simulink model "Python_GPUtesting_noPS"  (R2019a)
settings: Solver=FixedStepAuto  StartTime=0.0  StopTime=inf  FixedStep=1/ModelRate  RelTol=1e-3  EnableMultiTasking=on
undefined symbols (not defined in the file): DataRate, ModelRate, Ratio
libraries: xpcrtudplib x6, slrtlib x6, etargetslib x4
settings Model: SimulationMode=external  Creator=xugx0  LastModifiedBy=SI
settings SolverCC: ConcurrentTasks=on  AutoInsertRateTranBlk=on
settings DataIOCC: SaveFormat=StructureWithTime
settings OptimizationCC: BlockReduction=off  OptimizeBlockIOStorage=off  BufferReuse=off  GlobalBufferReuse=off  ExpressionFolding=off  LocalBlockOutputs=off  OptimizeDataStoreBuffers=off  BusAssignmentInplaceUpdate=off
settings DebuggingCC: ArithmeticOperatorsInVariantConditions=warning
settings HardwareCC: ProdBitPerPointer=32  ProdBitPerSizeT=32  ProdBitPerPtrDiffT=32  ProdLargestAtomicFloat=None  ProdWordSize=32  ProdLongLongMode=on  ProdHWDeviceType=Generic->32-bit x86 compatible
settings RTWCC: SystemTargetFile=slrt.tlc  TemplateMakefile=slrt_default_tmf  Description=Simulink Real-Time  CodeExecutionProfiling=on  RTWCompilerOptimization=on
settings CodeAppCC: StateflowObjectComments=on
settings SimulinkRealTimeCC: SupportVariableSizeSignals=on  PreserveStateflowLocalDataDimensions=off  RL32LogTETModifier=off  xPCConcurrentTasks=on

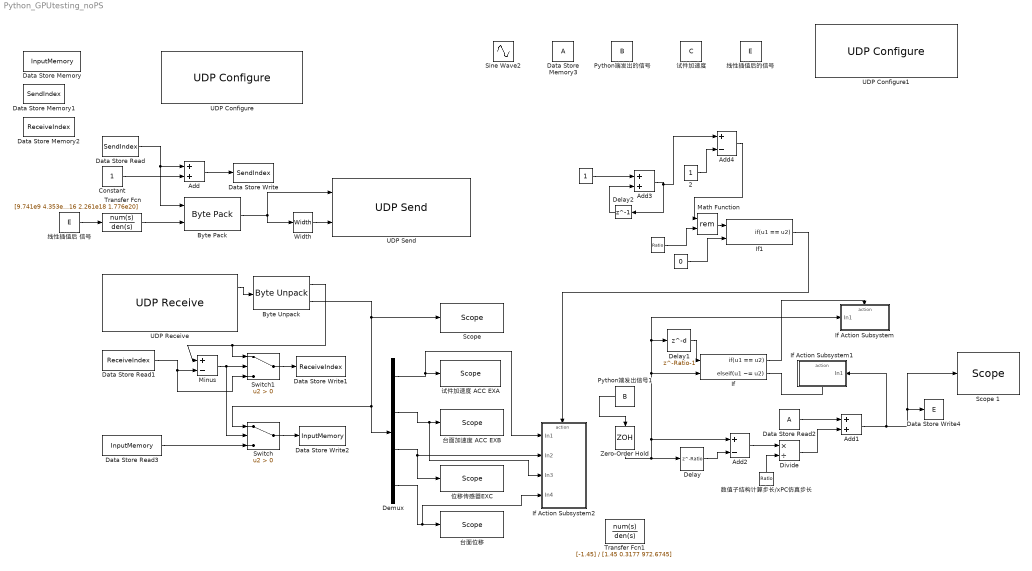
== system Python_GPUtesting_noPS ==
  " " : Constant  Value=Ratio
  " " : Constant  Value=0
  " " : Constant
  " 2" : Constant
  Add : Sum
  Add1 : Sum
  Add2 : Sum  Inputs=+-
  Add3 : Sum
  Add4 : Sum  Inputs=+-
  Byte Pack : etargetslib/Byte Pack  datatypes={'uint32','double'}  byteAlign=1
      settings: SourceProductName=MATLAB Coder
  Byte Unpack : etargetslib/Byte Unpack  dimensions={[1],[NumberOfInputSignals]}  datatypes={'uint32','double'}  byteAlign=1
      settings: SourceProductName=MATLAB Coder
  Constant : Constant  OutDataTypeStr=uint32
  Data Store Memory : DataStoreMemory  DataStoreName=InputMemory  ReadBeforeWriteMsg=warning  WriteAfterWriteMsg=warning  WriteAfterReadMsg=warning  InitialValue=InputMemInitV  ShowAdditionalParam=off
  Data Store Memory1 : DataStoreMemory  DataStoreName=SendIndex  ReadBeforeWriteMsg=warning  WriteAfterWriteMsg=warning  WriteAfterReadMsg=warning  ShowAdditionalParam=off  OutDataTypeStr=uint32
  Data Store Memory2 : DataStoreMemory  DataStoreName=ReceiveIndex  ReadBeforeWriteMsg=warning  WriteAfterWriteMsg=warning  WriteAfterReadMsg=warning  ShowAdditionalParam=off  OutDataTypeStr=uint32
  Data Store Memory3 : DataStoreMemory  ReadBeforeWriteMsg=warning  WriteAfterWriteMsg=warning  WriteAfterReadMsg=warning  ShowAdditionalParam=off
  Data Store Read : DataStoreRead  DataStoreName=SendIndex
  Data Store Read1 : DataStoreRead  DataStoreName=ReceiveIndex
  Data Store Read2 : DataStoreRead
  Data Store Read3 : DataStoreRead  DataStoreName=InputMemory
  Data Store Write : DataStoreWrite  DataStoreName=SendIndex
  Data Store Write1 : DataStoreWrite  DataStoreName=ReceiveIndex
  Data Store Write2 : DataStoreWrite  DataStoreName=InputMemory
  Data Store Write4 : DataStoreWrite  DataStoreName=E
  Delay : Delay  DelayLength=Ratio  InitialCondition=0
  Delay1 : Delay  DelayLength=Ratio-1  InitialCondition=0
  Delay2 : Delay  DelayLength=1  InitialCondition=0
  Demux : Demux
  Divide : Product  Inputs=*/
  If : If  NumInputs=2  IfExpression=u1 == u2  ElseIfExpressions=u1 ~= u2  ShowElse=off
  If Action Subsystem : Subsystem  TreatAsAtomicUnit=on
  If Action Subsystem1 : Subsystem  TreatAsAtomicUnit=on
  If Action Subsystem2 : Subsystem  TreatAsAtomicUnit=on
  If1 : If  NumInputs=2  IfExpression=u1 == u2  ShowElse=off
  Math Function : Math  Operator=rem  SaturateOnIntegerOverflow=on
  Minus : Sum  Inputs=+-
  Python端发出信号1 : DataStoreRead  DataStoreName=B
  Python端发出的信号 : DataStoreMemory  DataStoreName=B  ReadBeforeWriteMsg=warning  WriteAfterWriteMsg=warning  WriteAfterReadMsg=warning  ShowAdditionalParam=off
  "Scope " : slrtlib/Displays and Logging/Scope   scopeno=1  scopetype=Target  autostart=on  viewmode=Graphical sliding  formatstr='%15.6f'  grid=on  ylimits=[0,0]  nosamples=4000  noprepostsamples=0  interleave=1  triggermode=FreeRun  triggersignal=1  trigsignalfromport=off  triggerlevel=0.0  triggerslope=Either  triggerscope=1  triggersample=0  filename=data.dat  mode=Lazy  writesize=512  autorestart=off  dynamicfilemode=off  maxwritefilesize=512*1024^2
  Scope 1 : slrtlib/Displays and Logging/Scope   scopeno=2  scopetype=Target  autostart=on  viewmode=Graphical sliding  formatstr='%15.6f'  grid=on  ylimits=[0,0]  nosamples=4000  noprepostsamples=0  interleave=1  triggermode=FreeRun  triggersignal=1  trigsignalfromport=off  triggerlevel=0.0  triggerslope=Either  triggerscope=1  triggersample=0  filename=data.dat  mode=Lazy  writesize=512  autorestart=off  dynamicfilemode=off  maxwritefilesize=512*1024^2
  Sine Wave2 : Sin  Frequency=10  SampleTime=1/ModelRate
  Switch : Switch  Criteria=u2 > Threshold
  Switch1 : Switch  Criteria=u2 > Threshold
  Transfer Fcn : TransferFcn  Numerator=[9.741e9 4.353e13 1.087e16 2.844e18 1.773e20]  Denominator=[1.823e10 2.291e13 1.08e16 2.261e18 1.776e20]
  Transfer Fcn1 : TransferFcn  Numerator=[-1.45]  Denominator=[1.45 0.3177 972.6745]
  UDP Configure : xpcrtudplib/UDP Configure  Priority=-1  IpAddress=169.254.86.80  SubnetMask=255.255.0.0  Gateway=0.0.0.0  PciBus=5  PciSlot=Slot  PciFunction=0  ID=1  tune=0  disable=off  enableMulticast=off  MulticastIpAddress={}  MulticastMask={}
      settings: SourceProductName=Simulink Real-Time  SourceProductBaseCode=XP
  UDP Configure1 : xpcrtudplib/UDP Configure  Priority=-1  IpAddress=192.168.0.100  SubnetMask=255.255.255.0  Gateway=0.0.0.0  PciBus=4  PciSlot=Slot  PciFunction=0  ID=1  tune=0  disable=off  enableMulticast=off  MulticastIpAddress={}  MulticastMask={}
      settings: SourceProductName=Simulink Real-Time  SourceProductBaseCode=XP
  UDP Receive : xpcrtudplib/UDP Receive  ipAddressVal=169.254.86.80  localPort=LocalPort  rcvWidth=receiveLength  rcvFmAny=off  fmAddress=169.254.86.81  rcvMulticast=off  multicastAddress={}  maxUDPQueue=8  sampleTime=1/DataRate
      settings: SourceProductName=Simulink Real-Time
  UDP Send : xpcrtudplib/UDP Send  ipAddressVal=169.254.86.80  localPort=-1  toAddress=169.254.86.81  toPort=RemotePort  sampleTime=1/DataRate
      settings: SourceProductName=Simulink Real-Time  SourceProductBaseCode=XP
  Width : Width
  Zero-Order Hold : ZeroOrderHold  SampleTime=1/ModelRate
  位移传感器EXC : slrtlib/Displays and Logging/Scope   scopeno=6  scopetype=Target  autostart=on  viewmode=Graphical sliding  formatstr='%15.6f'  grid=on  ylimits=[0,0]  nosamples=4000  noprepostsamples=0  interleave=1  triggermode=FreeRun  triggersignal=1  trigsignalfromport=off  triggerlevel=0.0  triggerslope=Either  triggerscope=1  triggersample=0  filename=data.dat  mode=Lazy  writesize=512  autorestart=off  dynamicfilemode=off  maxwritefilesize=512*1024^2
  台面位移 : slrtlib/Displays and Logging/Scope   scopeno=7  scopetype=Target  autostart=on  viewmode=Graphical sliding  formatstr='%15.6f'  grid=on  ylimits=[0,0]  nosamples=4000  noprepostsamples=0  interleave=1  triggermode=FreeRun  triggersignal=1  trigsignalfromport=off  triggerlevel=0.0  triggerslope=Either  triggerscope=1  triggersample=0  filename=data.dat  mode=Lazy  writesize=512  autorestart=off  dynamicfilemode=off  maxwritefilesize=512*1024^2
  台面加速度 ACC EXB : slrtlib/Displays and Logging/Scope   scopeno=5  scopetype=Target  autostart=on  viewmode=Graphical sliding  formatstr='%15.6f'  grid=on  ylimits=[0,0]  nosamples=4000  noprepostsamples=0  interleave=1  triggermode=FreeRun  triggersignal=1  trigsignalfromport=off  triggerlevel=0.0  triggerslope=Either  triggerscope=1  triggersample=0  filename=data.dat  mode=Lazy  writesize=512  autorestart=off  dynamicfilemode=off  maxwritefilesize=512*1024^2
  数值子结构计算步长/xPC仿真步长 : Constant  Value=Ratio
  线性插值后 信号 : DataStoreRead  DataStoreName=E
  线性插值后的信号 : DataStoreMemory  DataStoreName=E  ReadBeforeWriteMsg=warning  WriteAfterWriteMsg=warning  WriteAfterReadMsg=warning  ShowAdditionalParam=off
  试件加速度 : DataStoreMemory  DataStoreName=C  ReadBeforeWriteMsg=warning  WriteAfterWriteMsg=warning  WriteAfterReadMsg=warning  ShowAdditionalParam=off
  试件加速度 ACC EXA : slrtlib/Displays and Logging/Scope   scopeno=4  scopetype=Target  autostart=on  viewmode=Graphical sliding  formatstr='%15.6f'  grid=on  ylimits=[0,0]  nosamples=4000  noprepostsamples=0  interleave=1  triggermode=FreeRun  triggersignal=1  trigsignalfromport=off  triggerlevel=0.0  triggerslope=Either  triggerscope=1  triggersample=0  filename=data.dat  mode=Lazy  writesize=512  autorestart=off  dynamicfilemode=off  maxwritefilesize=512*1024^2
  wires:
  Byte Pack/1 -> UDP Send/1, Width/1
  Width/1 -> UDP Send/2
  Switch/1 -> Data Store Write2/1
  Add/1 -> Data Store Write/1
  Constant/1 -> Add/2
  Data Store Read/1 -> Add/1, Byte Pack/1
  Minus/1 -> Switch1/2, Switch/2
  Data Store Read3/1 -> Switch/3
  UDP Receive/1 -> Byte Unpack/1
  Byte Unpack/1 -> Minus/1, Switch1/1
  Data Store Read1/1 -> Minus/2, Switch1/3
  Switch1/1 -> Data Store Write1/1
  Byte Unpack/2 -> Switch/1, Demux/1, "Scope "/1
  Add1/1 -> Scope 1/1, Data Store Write4/1, If Action Subsystem1/1(In1)
  Add2/1 -> Divide/1
  数值子结构计算步长/xPC仿真步长/1 -> Divide/2
  Divide/1 -> Add1/2
  Delay/1 -> Add2/2
  If/1 -> If Action Subsystem/Action
  If/2 -> If Action Subsystem1/Action
  Data Store Read2/1 -> Add1/1
  Zero-Order Hold/1 -> Add2/1, If/2, Delay1/1, If Action Subsystem/1(In1), Delay/1
  Delay1/1 -> If/1
  Python端发出信号1/1 -> Zero-Order Hold/1
  " "/1 -> Add3/1
  If1/1 -> If Action Subsystem2/Action
  Math Function/1 -> If1/1
  " "/1 -> Math Function/2
  " "/1 -> If1/2
  Add3/1 -> Add4/1, Delay2/1
  Delay2/1 -> Add3/2
  Demux/1 -> If Action Subsystem2/1(In1), 试件加速度 ACC EXA/1
  " 2"/1 -> Add4/2
  Add4/1 -> Math Function/1
  Demux/2 -> If Action Subsystem2/3(In3), 台面加速度 ACC EXB/1
  Demux/3 -> 位移传感器EXC/1, If Action Subsystem2/2(In2)
  Demux/4 -> If Action Subsystem2/4(In4), 台面位移/1
  Transfer Fcn/1 -> Byte Pack/2
  线性插值后 信号/1 -> Transfer Fcn/1

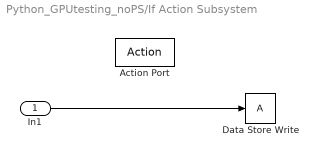
== system Python_GPUtesting_noPS/If Action Subsystem ==
  In1 : Inport
  Action Port : ActionPort  ActionPortLabel=if(u1 == u2)
  Data Store Write : DataStoreWrite
  wires:
  In1/1 -> Data Store Write/1

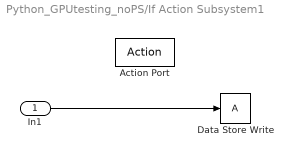
== system Python_GPUtesting_noPS/If Action Subsystem1 ==
  In1 : Inport
  Action Port : ActionPort  ActionPortLabel=elseif(u1 ~= u2)
  Data Store Write : DataStoreWrite
  wires:
  In1/1 -> Data Store Write/1

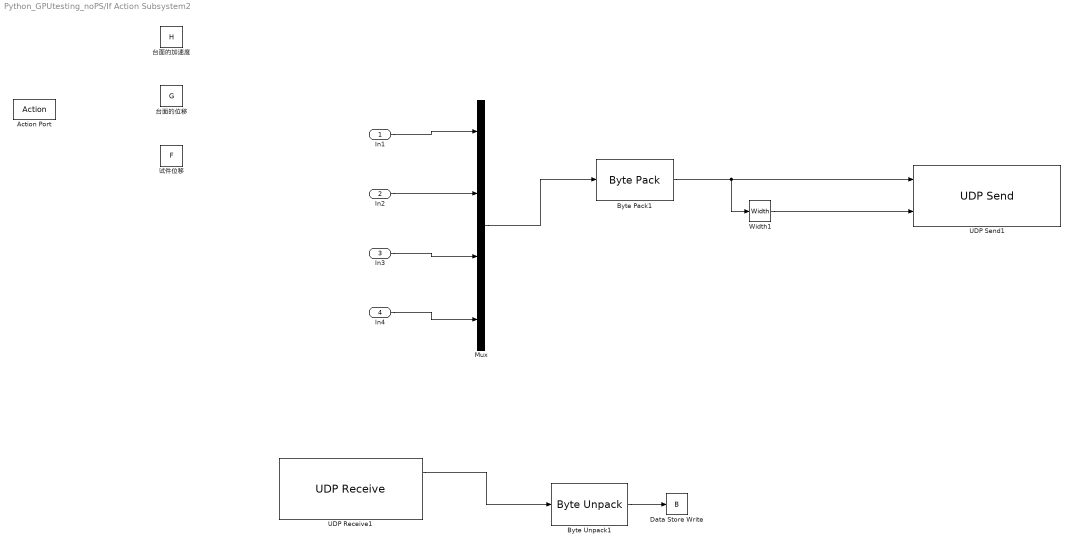
== system Python_GPUtesting_noPS/If Action Subsystem2 ==
  In1 : Inport
  In2 : Inport  Port=2
  In3 : Inport  Port=3
  In4 : Inport  Port=4
  Action Port : ActionPort  ActionPortLabel=if(u1 == u2)
  Byte Pack1 : etargetslib/Byte Pack  datatypes={'double'}  byteAlign=1
      settings: SourceProductName=MATLAB Coder
  Byte Unpack1 : etargetslib/Byte Unpack  dimensions={[1]}  datatypes={'double'}  byteAlign=1
      settings: SourceProductName=MATLAB Coder
  Data Store Write : DataStoreWrite  DataStoreName=B
  Mux : Mux
  UDP Receive1 : xpcrtudplib/UDP Receive  ipAddressVal=192.168.0.100  localPort=LocalPort  rcvWidth=8  rcvFmAny=off  fmAddress=192.168.0.101  rcvMulticast=off  multicastAddress={}  maxUDPQueue=8  sampleTime=1/DataRate
      settings: SourceProductName=Simulink Real-Time
  UDP Send1 : xpcrtudplib/UDP Send  ipAddressVal=192.168.0.100  localPort=-1  toAddress=192.168.0.101  toPort=RemotePort  sampleTime=1/DataRate
      settings: SourceProductName=Simulink Real-Time  SourceProductBaseCode=XP
  Width1 : Width
  台面的位移 : DataStoreMemory  DataStoreName=G  ReadBeforeWriteMsg=warning  WriteAfterWriteMsg=warning  WriteAfterReadMsg=warning  ShowAdditionalParam=off
  台面的加速度 : DataStoreMemory  DataStoreName=H  ReadBeforeWriteMsg=warning  WriteAfterWriteMsg=warning  WriteAfterReadMsg=warning  ShowAdditionalParam=off
  试件位移 : DataStoreMemory  DataStoreName=F  ReadBeforeWriteMsg=warning  WriteAfterWriteMsg=warning  WriteAfterReadMsg=warning  ShowAdditionalParam=off
  wires:
  UDP Receive1/1 -> Byte Unpack1/1
  Byte Unpack1/1 -> Data Store Write/1
  Width1/1 -> UDP Send1/2
  Byte Pack1/1 -> Width1/1, UDP Send1/1
  Mux/1 -> Byte Pack1/1
  In1/1 -> Mux/1
  In2/1 -> Mux/2
  In3/1 -> Mux/3
  In4/1 -> Mux/4
